simulink model "Simulink_VDP"  (R2022a)
settings: Solver=VariableStepAuto  StartTime=0.0  StopTime=100  FixedStep=ts  RelTol=1e-3
undefined symbols (not defined in the file or in its folder): ts
libraries: mpclib x1
settings Model: Creator=sergiovaneg  LastModifiedBy=sergiovaneg

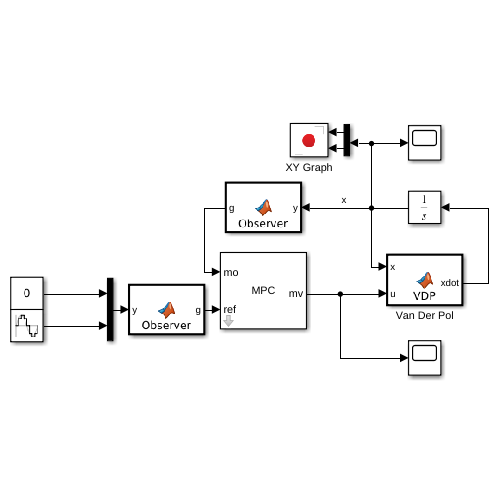
[thumbnail: Simulink's stored preview of the top-level diagram]
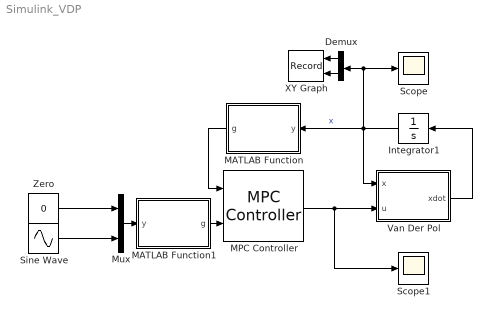
== system Simulink_VDP ==
  Demux : Demux  Outputs=2
  Integrator1 : Integrator
  MATLAB Function : MATLAB Function  TreatAsAtomicUnit=on
  MATLAB Function1 : MATLAB Function  TreatAsAtomicUnit=on
  MPC Controller : mpclib/MPC Controller  SCDEnableBlockLinearizationSpecification=on  mpcobj=mpcobj  is_multiple=0  enable_value=0  return_u0=off  updateMPCinCallerWorkspace=on  md_inport=off  mv_inport=off  uref_inport=off  return_cost=off  return_mvseq=off  return_qpstatus=off  return_xseq=off  return_state=off  return_ovseq=off  state_inport=off  umin_inport=off  umax_inport=off  ymin_inport=off  ymax_inport=off  cc_inport=off  ywt_inport=off  uwt_inport=off  duwt_inport=off  rhoeps_inport=off  pm_inport=off  MaximumP=10  HorizonChoice=FixedHorizon  n_ts=0.01  n_p=10  n_mv=1  n_md=0  n_ud=0  n_mo=1  n_uo=1  BlockDataType=double  SampleTimeInherited=off  switch_inport=off
  Mux : Mux  Inputs=2
  Scope : Scope
  Scope1 : Scope
  Sine Wave : Sin  Frequency=pi  Samples=100  SampleTime=ts
  Van Der Pol : MATLAB Function  TreatAsAtomicUnit=on
  XY Graph : Record  FileSettingsInternal="{\"entries\":[{\"content\":{\"excelSettings\":{\"content\":{},\"type\":\"Streamout.ExcelSettings\"}},\"type\":\"Streamout.FileSettingStorage\",\"uuid\":\"321c7dc2-94c2-4a1e-b015-5c3c2f0bf0e9\"}],\"packageUris\":[\"http://schema.mathworks.com/mf0/streamout_blocks/R2020a\"],\"version\":\"1.0\"}"  Layout=[1 1]  SignalsInternal="{\"entries\":[{\"content\":{\"signals\":[{\"content\":{\"blockPath\":[\"Simulink_VDP/XY Graph\"],\"channel\":[],\"dimensions\":[1],\"domain\":\"Simulink_VDP/XY Graph\",\"lineColor\":\"#a2142f\",\"plots\":[1],\"port\":1,\"sid\":[],\"signalID\":28,\"signalName\":\"XY Graph:1\"},\"type\":\"RecordBlkView.Signal\",\"uuid\":\"0383c83c-9483-48cb-bce9-8902a680ab1d\"},{\"content\":{\"blockPath\":[\"Simulink_VDP/XY Graph\"],\"channel\":[],\"dimensions\":[1],\"domain\":\"Simulink_VDP/XY Graph\",\"lineColor\":\"#139fff\",\"plots\":[1],\"port\":2,\"sid\":[],\"signalID\":31,\"signalName\":\"XY Graph:2\"},\"type\":\"RecordBlkView.Signal\",\"uuid\":\"256aacad-c8e4-4715-808c-6d6bf8b71f59\"}]},\"type\":\"RecordBlkView.InputSignals\",\"uuid\":\"f9c25911-d564-4c04-8c45-c85ce707bc4b\"}],\"packageUris\":[\"http://schema.mathworks.com/mf0/streamout_blocks/R2020a\"],\"version\":\"1.0\"}"  VisualizationBindings="{\"xyplotplugin\":{\"info\":[{\"series\":[{\"bindingParametersList\":[{\"parameter\":\"X-Axis\",\"signalID\":28,\"signalName\":\"XY Graph:1\"},{\"parameter\":\"Y-Axis\",\"signalID\":31,\"signalName\":\"XY Graph:2\"}],\"seriesID\":63274}],\"subplotID\":1}]}}"  CompatibilityTag=XY
  Zero : Constant  Value=0  OutDataTypeStr=Inherit: Inherit via back propagation
  wires:
  Van Der Pol/1(xdot) -> Integrator1/1
  Integrator1/1 -> MATLAB Function/1(y), Scope/1, Demux/1, Van Der Pol/1(x)  "x"
  MPC Controller/1 -> Scope1/1, Van Der Pol/2(u)
  Zero/1 -> Mux/1
  Sine Wave/1 -> Mux/2
  MATLAB Function/1(g) -> MPC Controller/1
  Mux/1 -> MATLAB Function1/1(y)
  MATLAB Function1/1(g) -> MPC Controller/2
  Demux/1 -> XY Graph/1
  Demux/2 -> XY Graph/2

== matlab function Simulink_VDP/Van Der Pol ==
  data: x input; u input; xdot output
function xdot = VDP(x,u)
xdot = zeros(2,1);
xdot(1)=2*x(2);
xdot(2)=-0.8*x(1)+2*x(2)-10*(x(1)^2)*x(2)+u;

== matlab function Simulink_VDP/MATLAB Function1 ==
  data: y input; g output
function g = Observer(y)
    n = size(X0,1);
    N = size(X0,2);
    g = [y;
        zeros(N,1)];

    for i=1:N
        x0 = X0(:,i);
        g(i+n,:) = vecnorm(y-x0).*log(vecnorm(y-x0).^vecnorm(y-x0));    
    end

== matlab function Simulink_VDP/MATLAB Function ==
  data: y input; g output
function g = Observer(y)
    n = size(X0,1);
    N = size(X0,2);
    g = [y;
        zeros(N,1)];

    for i=1:N
        x0 = X0(:,i);
        g(i+n,:) = vecnorm(y-x0).*log(vecnorm(y-x0).^vecnorm(y-x0));    
    end
